simulink library "elements"  (Simulink 8.5)
settings: Solver=ode45  SolverMode=SingleTasking  StartTime=0.0  StopTime=10.0  RelTol=1e-3
values from neighbouring files (symbols this model uses):
  n = abs(fix(dif/360))    [DE_12.m]
undefined symbols (not defined in the file or in its folder): aux, b, Den, den, dx, flagc, in, k, m, minx, nin, num, Num
settings Model: Creator=PC  LastModifiedBy=PC

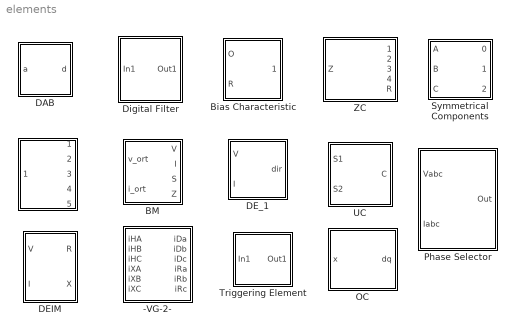
== system elements ==
  " " : Subsystem  mask(Digital Fourier Transform){fo=60, window_size=20, harmonic=[1 2 3 4 5]}
      mask prompts: fo "Fundamental frequency (Hz)"; window_size "Window size"; harmonic "Requested harmonics (up to five harmonics)"
      mask help: Captures the data window of a sampled signal and computes the phasors (magnitude and angle) of up to 5 selected harmonics including the dc component. The fundamental frequency, the data window size as well as the array that specify the requested harmonic must be defined.
      mask Display: disp('DFT')
  "  DE_1" : Subsystem  mask(Directional Element 1){alpha=10, beta=170, fs=20*60}
      mask prompts: alpha "Angle alpha [deg]"; beta "Angle Beta [deg]"; fs "Sampling frecuency (Hz):"
      mask help: This block has two phasor inputs: voltage and current. The operating characteristic is defined by two angles. The output is 1 when the current phasor falls into the operating characteristic.
      mask init:
      | DE_11;
      mask Display: plot([0.2 0.8],[0.5 0.5],[0.5 0.6],[0.5 0.8],[0.5,xalpha],[0.5,yalpha],[0.5,xbeta],[0.5,ybeta]);
  -VG-2- : Subsystem  mask(Transformer Masked Block){trtype=wye - wye, vector=0, Vh=345000, Vx=389800, nCTH=400, nCTX=400}
      mask prompts: trtype "Type of Transformer"; vector "Vector Group"; Vh "Primary Voltage"; Vx "Secondary Voltage"; nCTH "CT Ratio of H"; nCTX "CT Ratio of X"
      mask help: Captures the instantaneous values of six phase currents and computes the differential and restraining currents of a 2-winding transformer. The type of transformer, vector group, voltages and CT ratios for the primary and secondary sides of the transformers must be specified. Selection of type of transformer and vector group.
      mask init:
      | vg_20;
      mask TypeOptions trtype: wye - delta | delta - wye | wye - wye | delta - delta
      mask TypeOptions vector: 0 | 1 | 3 | 5 | 6 | 7 | 9 | 11
      mask Display: disp(icon)
  BM : Subsystem  mask(BM){tpostv=none, plenv=4, tposti=none, pleni=4, tposts=none, plens=4, tpostz=none, plenz=4}
      mask prompts: tpostv "Type of post filtration for voltage"; plenv "Width of post filtration data window for voltage"; tposti "Type of post filtration for current"; pleni "Width of post filtration data window for current"; tposts "Type of post filtration for power"; plens "Width of post filtration data window for power"; tpostz "Type of post filtration for impedance"; plenz "Width of post filtration data window for impedance"
      mask help: This block is fed by the orthogonal components of the voltage and current signals (amplitude and angle in degrees). Its outputs are the current and voltage amplitudes, active and reactive powers and impedance components. The options include type of post-filtering (none, mean and median) with adjustable window length.
      mask TypeOptions tpostv: none | mean | median
      mask TypeOptions tposti: none | mean | median
      mask TypeOptions tposts: none | mean | median
      mask TypeOptions tpostz: none | mean | median
  Bias Characteristic : Subsystem  mask(Bias Characteristic){BC=[ 0 0;1 0.5 ;3 0.8; 5 4; 7 4.2 ; 8 4.22], fs=60*20}
      mask prompts: BC "Bias characteristic"; fs "Sampling frequency [samples per cycle]"
      mask help: Compares its two input signals using a bias characteristic. This characteristic is defined point-by-point.
      mask init:
      | bc2
      mask Display:
      | plot([xo xo],[yo y1]);
      | plot([xo x1],[yo yo]);
      | 
      | 
      | plot(R,O);
  DAB : Subsystem  mask(Data Adquisition Board){filter=off, approx=Bessel, order=2, numerator=[], denominator=[], freq=180, resdis=off, vertres=12, xmax=10, winsize=40, G=1.0, fs=60*40}
      mask prompts: filter "Disable Analog Filter"; approx "Filter approximation"; numerator "Free expression filter: numerator(descending order of s)"; denominator "Free expression filter: denominator:"; freq "Cut-off frequency"; resdis "Disable Vertical Resolution"; vertres "Vertical Resolution: No. of bits"; xmax "Vertical Resolution: signal range"; winsize "Window size"; G "Gain"; fs "Sampling frequency"
      mask help: Performs analog filtering, signal conditioning and sampling. A single signal is the input, a buffer with the signal samples is the output. The options include analog filter enable/disable switch, type, order and cut-off frequency of the analog filter, conditioning gain, sampling frequency, number of bits, the length of the buffer.
      mask init:
      | dab1
      mask TypeOptions approx: Bessel | Tschebyscheff | Butterworth | free expression
      mask TypeOptions order: 2 | 3 | 4
      mask TypeOptions vertres: 8 | 12 | 16
      mask Display: disp('DAB')
  DEIM : Subsystem  mask(Differential Equation based  Impedance Measurement){type_pre=none, meth_sol=The least square method, num_meth=Euler, type_post=none, N=10, d=10, m=5, p=10, f=20*60, f1=60}
      mask prompts: type_pre "Type of pre-processing"; meth_sol "Type of methods for solution"; num_meth "Type of numerical integration/differentation method"; type_post "Type of post processing filters"; N "Size of input window"; d "Size of data window for the least square method"; m "Size of data window for succesive samples method"; p "Size of data window for post processing filters"; f "Sampling frequency [Hz]"; f1 "Fundamental frequency"
      mask help: Measures the impedance based on the differential equation approach. The options include pre- and post-filtering, the method of differentiation, and the method of generating the missing equation.
      mask init:
      | N1=f/f1;
      | Tsamp=1/f;
      | Tw=(N1+1)*Tsamp;
      | deim1
      mask TypeOptions type_pre: none | quarter Fourier filter | half Fourier filter | quarter Walsh filter | half Walsh filter
      mask TypeOptions meth_sol: Two points in time dislocated by m samples | The least square method
      mask TypeOptions num_meth: Euler | Trapezoidal rule
      mask TypeOptions type_post: none | mean filter | median filter
  Digital Filter : Subsystem  mask(Digital Filter){FilterType=Chebyshev, PassType=lowpass, IIROrder=2, fs=32*60, CutFre=[300], DataWindow=32, winsize=1, frequency0=60, FreeZformNum=[0  1 ], FreeZformDen=[ 1 ]}
      mask prompts: FilterType "Filter Type"; PassType "Pass Type"; IIROrder "IIR Filter Order"; fs "Sampling Frequency (Hz)"; CutFre "Cut-off Frequency (Hz)"; DataWindow "Data Window for FIR filters"; winsize "Output data window"; frequency0 "Fundamental Frequency (Hz)"; FreeZformNum "Numerator of the free expression filter"; FreeZformDen "Denominator of the free expression filter"
      mask help: This block captures the data window of a sampled signal and filters the signal. The predefined filters include Fourier and Walsh functions. The free expression filters may also be used.
      mask init:
      | df1
      mask TypeOptions FilterType: Fourier_Sine | Fourier_Cosine | Walsh1 | Walsh2 | Walsh3 | Walsh4 | Butterworth | Bessel | Chebyshev | Free expression
      mask TypeOptions PassType: lowpass | highpass | bandpass | bandstop
      mask TypeOptions IIROrder: 1 | 2 | 3
      mask Display: disp(DIFI);
  OC : Subsystem  mask(Orthogonal Components){tfilt=User Defined, rfilt=[ ], ifilt=[ ], tlen=full, N1=40}
      mask prompts: tfilt "Type of filter:"; rfilt "Direct filter"; ifilt "Quadrature filter"; tlen "Type of data window"; N1 "Number of samples per cycle:"
      mask help: The block captures the data window of a sampled signal and computes the orthogonal components of the signal, i.e. amplitude and angle. The pre-defined filters include Fourier and Walsh functions. The free expression filters may also be used. Note: The type of data window affects only the Fourier filter.
      mask init:
      | oc2;
      mask TypeOptions tfilt: Fourier | Walsh | User Defined
      mask TypeOptions tlen: half | full
      mask Display: disp(DIFI);
  Phase Selector : Subsystem  mask(Phase Selection){THI=3, THV=3, THZ=3, THG=0.5, METHOD=Current and Voltage and Impedance}
      mask prompts: THI "Threshold for Current"; THV "Threshold for Voltage"; THZ "Threshold for Impedance"; THG "Threshold for zero-sequence current"
      mask help: The inputs of this block are the orthogonal components of the three-phase voltage and currents. It recognizes the type of fault based on the inputs. The methods include current-only, voltage-only and combined signal classification. The thresholds for the current, voltage and impedance must be specified accordingly.
      mask init:
      | ps1
      mask TypeOptions METHOD: Current | Voltage | Impedance | Current and Voltage | Current or Voltage | Current and Impedance | Current or Impedance | Voltage and Impedance | Voltage or Impedance | Current and Voltage and Impedance | Current or Voltage or Impedance
      mask Display: disp(icon)
  Symmetrical Components : Subsystem  mask(Symmetrical Components){ortho_instant=Orthogonal, powerfre=60, samplefre=1200}
      mask prompts: ortho_instant "Orthogonal or Instantaneous"; powerfre "Signal Fundamental Frequency"; samplefre "Sampling Frequency (Hz)"
      mask help: The inputs of the block are the three phase signals and the outputs are the symmetrical components. The inputs can be instantaneous (3 inputs) or orthogonal components i.e. magnitudes and angles of the signals (6 inputs). The outputs represent the signal type specificied for inputs.
      mask init:
      | sc2;
      mask TypeOptions ortho_instant: Orthogonal | Instantaneous
      mask Display: disp(DIFI);
  Triggering Element : Subsystem  mask(TR){METHOD=Sample to sample, TH=.5, p=1, q=4, SF=60*80, SN=80, ti=0.02}
      mask prompts: TH "Threshold"; p "Activating counter"; q "Deactivating counter"; SF "Sampling frecuency"; SN "Window size"; ti "Start-up time"
      mask help: This block acts as a fault detector. The implemented methods include sample by sample checking, cycle by cycle checking, instantaneous value and amplitude as the triggering parameter. The options include also the limits for the set and re-set counters.
      mask TypeOptions METHOD: Value | Sample to sample | Cycle to cycle
      mask Display: disp('TR')
  UC : Subsystem  mask(Universal Comparator){type0=Signal-Threshold, sign=<, Ipickup=3, k1=1, type1=Time defined, type3=integration, k=10, fs=40*60}
      mask prompts: type0 "Type of comparison"; Ipickup "Pick-up value:"; k1 "Ratio of reset to pick-up:"; type1 "Type of Time dependency"; type3 "I-t emulation method"; k "Time parameter (seconds):"; fs "Sampling frequency (Hz):"
      mask help: This block is fed by two signals and does comparisons of three types: signal-to-signal, signal-to-threshold and signal-to-time. The options include the sign of the comparison, pick-up to re-set ratio, and the way of emulating the steady-state current characteristic.
      mask init:
      | uc0;
      mask TypeOptions type0: Signal-Threshold | Signal-Signal | Signal-Time
      mask TypeOptions sign: > | <
      mask TypeOptions type1: Time defined | Standard Inverse | Very Inverse | Extra Inverse | RI Inverse | Long Time Inverse
      mask TypeOptions type3: Present value | integration
      mask Display:
      | disp(icon);
      | plot(current,time);
  "ZC   " : Subsystem  mask(Zone Comparator){typez=Free expression, z1=[0 0 ;1 0; 1 1; 0.5 1], z2=[0 0; 2 0; 2 2; 1 2], z3=[0 0; 3 0; 4 3 ;1 3], z4=[0 0; 4 0; 5 4; 1 5], zr=[0 0; -1 0; -1 -1; 0 -1], fs=4*60}
      mask prompts: typez "shape"; z1 "Zone 1"; z2 "Zone 2"; z3 "Zone 3"; z4 "Zone 4"; zr "Reverse Zone"; fs "Sampling frecuency (Hz):"
      mask help: This block performs the zone comparison. Its inputs are the resistance and reactance signals. Four forward and one backward zones are implemented. The output that corresponds to the zone where the impedance is located is set to one while the rest of the outputs are zero Either the mho or free expression characteristics may be set. For the mho characteristic, the zones are defined by specifying the center of each circle (all the circles are tangent to the origin). For the free expression, arrays with consecutive vertices specify the polygons for each zone.
      mask init:
      | zc1;
      mask TypeOptions typez: Mho characteristic | Free expression
      mask Display:
      | plot(x1(:,1),x1(:,2));
      | plot(x2(:,1),x2(:,2));
      | plot(x3(:,1),x3(:,2));
      | plot(x4(:,1),x4(:,2));
      | plot(xr(:,1),xr(:,2));

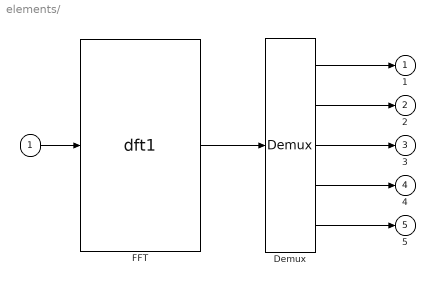
== system elements/  ==
  " " : Inport
  Demux : Demux  Outputs=5
  FFT : S-Function  FunctionName=dft1  Parameters=window_size, fo,harmonic
  "1 " : Outport  InitialOutput=0
  "2 " : Outport  Port=2  InitialOutput=0
  "3 " : Outport  Port=3  InitialOutput=0
  "4 " : Outport  Port=4  InitialOutput=0
  "5 " : Outport  Port=5  InitialOutput=0
  wires:
  FFT/1 -> Demux/1
  Demux/1 -> "1 "/1
  Demux/2 -> "2 "/1
  Demux/3 -> "3 "/1
  Demux/5 -> "5 "/1
  Demux/4 -> "4 "/1
  " "/1 -> FFT/1

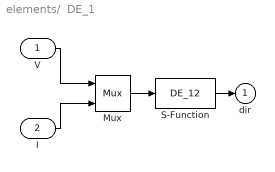
== system elements/  DE_1 ==
  V : Inport
  I : Inport  Port=2
  Mux : Mux  Inputs=2
  S-Function : S-Function  FunctionName=DE_12  Parameters=alpha,beta,fs
  dir : Outport  InitialOutput=0
  wires:
  S-Function/1 -> dir/1
  Mux/1 -> S-Function/1
  V/1 -> Mux/1
  I/1 -> Mux/2

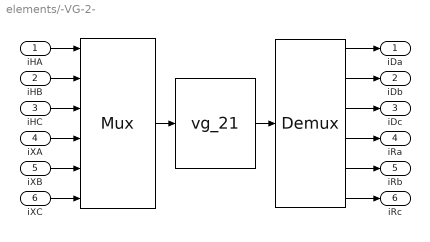
== system elements/-VG-2- ==
  iHA : Inport
  iHB : Inport  Port=2
  iHC : Inport  Port=3
  iXA : Inport  Port=4
  iXB : Inport  Port=5
  iXC : Inport  Port=6
  " " : Mux  Inputs=6
  "  " : Demux  Outputs=6
  "    " : S-Function  FunctionName=vg_21  Parameters=trtype,vector,Vh,Vx,nCTH,nCTX
  iDa : Outport  InitialOutput=0
  iDb : Outport  Port=2  InitialOutput=0
  iDc : Outport  Port=3  InitialOutput=0
  iRa : Outport  Port=4  InitialOutput=0
  iRb : Outport  Port=5  InitialOutput=0
  iRc : Outport  Port=6  InitialOutput=0
  wires:
  " "/1 -> "    "/1
  "    "/1 -> "  "/1
  "  "/1 -> iDa/1
  iHA/1 -> " "/1
  "  "/2 -> iDb/1
  iHB/1 -> " "/2
  "  "/3 -> iDc/1
  iHC/1 -> " "/3
  "  "/4 -> iRa/1
  iXA/1 -> " "/4
  "  "/5 -> iRb/1
  iXB/1 -> " "/5
  "  "/6 -> iRc/1
  iXC/1 -> " "/6

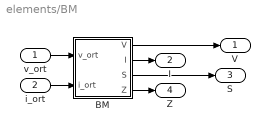
== system elements/BM ==
  v_ort : Inport
  i_ort : Inport  Port=2
  BM : Subsystem
  V : Outport  InitialOutput=0
  I : Outport  Port=2  InitialOutput=0
  S : Outport  Port=3  InitialOutput=0
  Z : Outport  Port=4  InitialOutput=0
  wires:
  BM/1(V) -> V/1
  v_ort/1 -> BM/1(v_ort)
  BM/2(I) -> I/1
  BM/3(S) -> S/1
  i_ort/1 -> BM/2(i_ort)
  BM/4(Z) -> Z/1

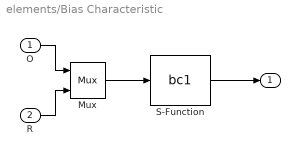
== system elements/Bias Characteristic ==
  O : Inport
  R : Inport  Port=2
  Mux : Mux  Inputs=2
  S-Function : S-Function  FunctionName=bc1  Parameters=BC,fs
  " " : Outport
  wires:
  Mux/1 -> S-Function/1
  R/1 -> Mux/2
  O/1 -> Mux/1
  S-Function/1 -> " "/1

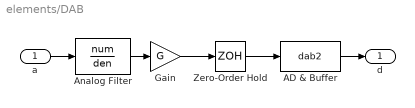
== system elements/DAB ==
  a : Inport
  AD & Buffer : S-Function  FunctionName=dab2  Parameters=winsize,fs,dx,resdis
  Analog Filter : TransferFcn  Numerator=num  Denominator=den
  Gain : Gain  Gain=G  SaturateOnIntegerOverflow=on  OutDataTypeStr=Inherit: Same as input  ParamDataTypeStr=Inherit: Same as input
  Zero-Order Hold : ZeroOrderHold  SampleTime=1/fs
  d : Outport  InitialOutput=[zeros(winsize,1)]
  wires:
  Analog Filter/1 -> Gain/1
  Gain/1 -> Zero-Order Hold/1
  Zero-Order Hold/1 -> AD & Buffer/1
  a/1 -> Analog Filter/1
  AD & Buffer/1 -> d/1

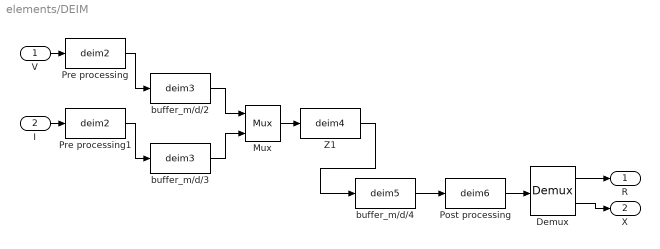
== system elements/DEIM ==
  V : Inport
  I : Inport  Port=2
  Demux : Demux  Outputs=2
  Mux : Mux  Inputs=2
  Post processing : S-Function  FunctionName=deim6  Parameters=Tsamp,in,type_post
  Pre processing : S-Function  FunctionName=deim2  Parameters=N,nin,Tsamp,Tw,type_pre
  Pre processing1 : S-Function  FunctionName=deim2  Parameters=N,nin,Tsamp,Tw,type_pre
  Z1 : S-Function  FunctionName=deim4  Parameters=Tsamp,k,meth_sol,num_meth
  buffer_m/d/2 : S-Function  FunctionName=deim3  Parameters=Tsamp,nin,k
  buffer_m/d/3 : S-Function  FunctionName=deim3  Parameters=Tsamp,nin,k
  buffer_m/d/4 : S-Function  FunctionName=deim5  Parameters=Tsamp,in
  R : Outport
  X : Outport  Port=2
  wires:
  Z1/1 -> buffer_m/d/4/1
  I/1 -> Pre processing1/1
  V/1 -> Pre processing/1
  Demux/1 -> R/1
  Demux/2 -> X/1
  buffer_m/d/4/1 -> Post processing/1
  Post processing/1 -> Demux/1
  Mux/1 -> Z1/1
  buffer_m/d/2/1 -> Mux/1
  buffer_m/d/3/1 -> Mux/2
  Pre processing1/1 -> buffer_m/d/3/1
  Pre processing/1 -> buffer_m/d/2/1

== system elements/Digital Filter ==
  In1 : Inport
  " FIR and IIR Filters " : DiscreteFilter  Numerator=Num  Denominator=Den  SampleTime=1/fs
  S-Function : S-Function  FunctionName=df2  Parameters=winsize,fs
  Out1 : Outport  InitialOutput=0
  wires:
  In1/1 -> " FIR and IIR Filters "/1
  " FIR and IIR Filters "/1 -> S-Function/1
  S-Function/1 -> Out1/1

== system elements/OC ==
  note: v_ort is
      | a complex number
  note: v(t) is a vector
      | with width N1
  x : Inport
  OC filter : S-Function  FunctionName=oc1  Parameters=tfilt, rfilt, ifilt, tlen, N1
  dq : Outport  InitialOutput=0
  wires:
  OC filter/1 -> dq/1
  x/1 -> OC filter/1

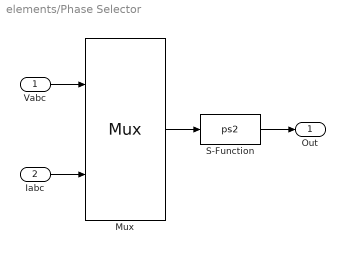
== system elements/Phase Selector ==
  Vabc : Inport
  Iabc : Inport  Port=2
  Mux : Mux  Inputs=2
  S-Function : S-Function  FunctionName=ps2  Parameters=THI, THV, THZ, THG,METHOD
  Out : Outport  InitialOutput=0
  wires:
  Vabc/1 -> Mux/1
  Mux/1 -> S-Function/1
  S-Function/1 -> Out/1
  Iabc/1 -> Mux/2

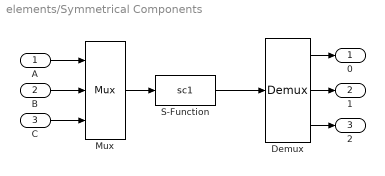
== system elements/Symmetrical Components ==
  A : Inport
  B : Inport  Port=2
  C : Inport  Port=3
  Demux : Demux  Outputs=3
  Mux : Mux  Inputs=3
  S-Function : S-Function  FunctionName=sc1  Parameters=ortho_instant,powerfre,samplefre
  0 : Outport  InitialOutput=0
  1 : Outport  Port=2  InitialOutput=0
  2 : Outport  Port=3  InitialOutput=0
  wires:
  Mux/1 -> S-Function/1
  C/1 -> Mux/3
  B/1 -> Mux/2
  A/1 -> Mux/1
  Demux/3 -> 2/1
  Demux/2 -> 1/1
  Demux/1 -> 0/1
  S-Function/1 -> Demux/1

== system elements/Triggering Element ==
  In1 : Inport
  S-Function : S-Function  FunctionName=tr1  Parameters=TH,p,q,SF,SN,METHOD,ti
  Out1 : Outport  InitialOutput=0
  wires:
  S-Function/1 -> Out1/1
  In1/1 -> S-Function/1

== system elements/UC ==
  S1 : Inport
  S2 : Inport  Port=2
  Mux : Mux  Inputs=2
  S-Function : S-Function  FunctionName=uc1  Parameters=k,k1,aux,Ipickup,fs
  C : Outport  InitialOutput=0
  wires:
  S2/1 -> Mux/2
  S1/1 -> Mux/1
  Mux/1 -> S-Function/1
  S-Function/1 -> C/1

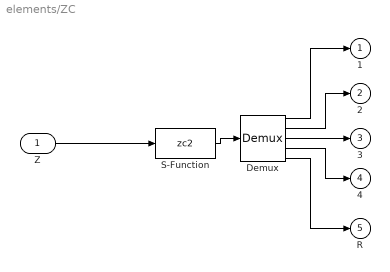
== system elements/ZC    ==
  Z : Inport
  Demux : Demux  Outputs=5
  S-Function : S-Function  FunctionName=zc2  Parameters=z1,z2,z3,z4,zr,typez,fs,n,minx,flagc,m,b
  1 : Outport  InitialOutput=0
  2 : Outport  Port=2  InitialOutput=0
  3 : Outport  Port=3  InitialOutput=0
  4 : Outport  Port=4  InitialOutput=0
  R : Outport  Port=5  InitialOutput=0
  wires:
  S-Function/1 -> Demux/1
  Demux/1 -> 1/1
  Demux/2 -> 2/1
  Demux/3 -> 3/1
  Demux/4 -> 4/1
  Z/1 -> S-Function/1
  Demux/5 -> R/1

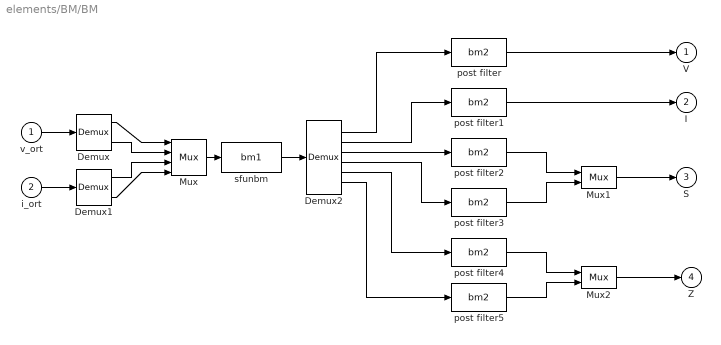
== system elements/BM/BM ==
  v_ort : Inport
  i_ort : Inport  Port=2
  Demux : Demux  Outputs=2
  Demux1 : Demux  Outputs=2
  Demux2 : Demux  Outputs=6
  Mux : Mux
  Mux1 : Mux  Inputs=2
  Mux2 : Mux  Inputs=2
  post filter : S-Function  FunctionName=bm2  Parameters=tpostv, plenv
  post filter1 : S-Function  FunctionName=bm2  Parameters=tposti, pleni
  post filter2 : S-Function  FunctionName=bm2  Parameters=tposts, plens
  post filter3 : S-Function  FunctionName=bm2  Parameters=tposts, plens
  post filter4 : S-Function  FunctionName=bm2  Parameters=tpostz, plenz
  post filter5 : S-Function  FunctionName=bm2  Parameters=tpostz, plenz
  sfunbm : S-Function  FunctionName=bm1
  V : Outport  InitialOutput=0
  I : Outport  Port=2  InitialOutput=0
  S : Outport  Port=3  InitialOutput=0
  Z : Outport  Port=4  InitialOutput=0
  wires:
  post filter5/1 -> Mux2/2
  post filter4/1 -> Mux2/1
  post filter3/1 -> Mux1/2
  post filter2/1 -> Mux1/1
  Mux2/1 -> Z/1
  Mux1/1 -> S/1
  post filter1/1 -> I/1
  post filter/1 -> V/1
  Mux/1 -> sfunbm/1
  Demux/1 -> Mux/1
  Demux1/1 -> Mux/3
  Demux1/2 -> Mux/4
  sfunbm/1 -> Demux2/1
  Demux/2 -> Mux/2
  v_ort/1 -> Demux/1
  i_ort/1 -> Demux1/1
  Demux2/3 -> post filter2/1
  Demux2/2 -> post filter1/1
  Demux2/1 -> post filter/1
  Demux2/4 -> post filter3/1
  Demux2/5 -> post filter4/1
  Demux2/6 -> post filter5/1
